simulink model "BSPK_Sound"  (R2024b)
settings: Solver=VariableStepAuto  StartTime=0.0  StopTime=5.5  RelTol=1e-3
libraries: commdigbbndpm3 x2, simulink x2, commchan3 x1, commsink2 x1, dspvision x1, dspsnks4 x1
settings Model: Creator=sarriola  LastModifiedBy=RomaW11
settings SolverCC: AlgebraicLoopSolver=TrustRegion
settings DataIOCC: ReturnWorkspaceOutputs=off
settings OptimizationCC: LifeSpan=inf
settings DebuggingCC: UnconnectedInputMsg=warning  UnconnectedOutputMsg=warning  UnconnectedLineMsg=warning  SFExecutionAtInitializationDiag=none  ArithmeticOperatorsInVariantConditions=warning
settings ModelReferenceCC: EnableRefExpFcnMdlSchedulingChecks=on
settings SFSimCC: SimUseLocalCustomCode=off  CustomCodeUndefinedFunction=UseInterfaceOnly
settings RTWCC: RTWUseLocalCustomCode=off  GPUComputeCapability=3.5
settings CodeAppCC: StateflowObjectComments=on

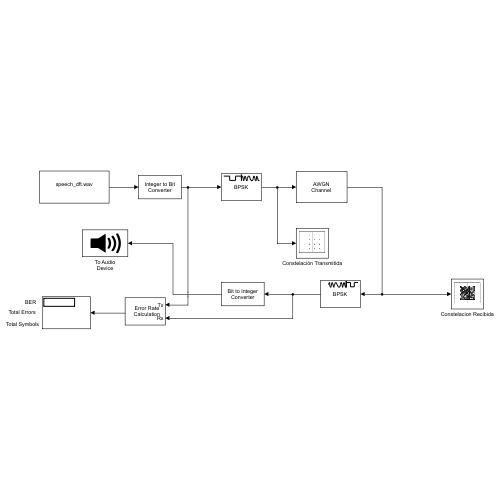
[thumbnail: Simulink's stored preview of the top-level diagram]
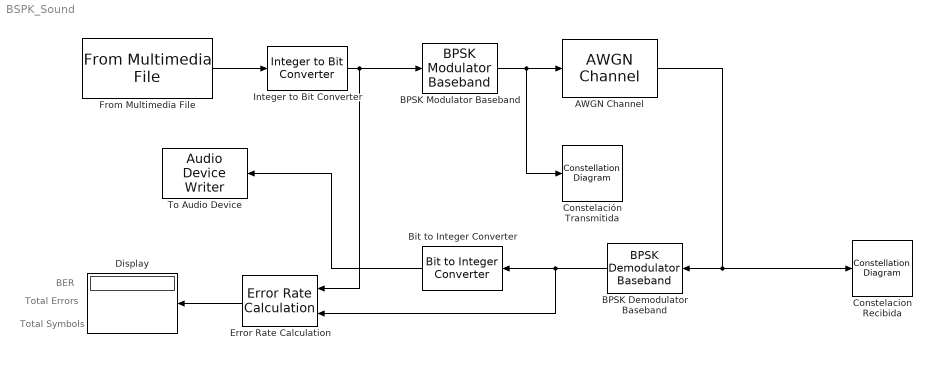
== system BSPK_Sound ==
  note: Total Symbols
  note: Total Errors
  note: BER
  AWGN Channel : commchan3/AWGN Channel  LegacyMode=on  NoiseMethod="Signal to noise ratio  (SNR)"  noiseMode="Signal to noise ratio  (SNR)"  EbNo=60  EsNo=10  SNR=30  BitsPerSymbol=1  SignalPower=1  SamplesPerSymbol=1  SymbolPeriod=1  VarianceSource=Parameter  Variance=1  RandomStream=Global stream  Seed=67  SimulateUsing=Code generation
  BPSK Demodulator Baseband : commdigbbndpm3/BPSK Demodulator Baseband  DecType=Hard decision  VarSource=Dialog  Variance=1  Ph=0  outDtype=int16  derotateFactorWordLen=16  derotateFactorDataTypeStr=Inherit: Same word length as input  derotateFactorLastDataTypeStr=Inherit: Same word length as input
  BPSK Modulator Baseband : commdigbbndpm3/BPSK Modulator Baseband  Ph=0  outDtype=double  outWordLen=16  outUDDataType=sfix(16)  outFracLenMode=Best precision  outFracLen=15  outDataTypeStr=double  outLastDataTypeStr=double
  Bit to Integer Converter : simulink/Logic and Bit Operations/Bit to Integer Converter  nbits=16  bitOrder=MSB first  signedOutputValues=Signed  outDtype=int16  outDtypeSigned=int16
      settings: LibrarySourceBlock=|
      | commutil2/Bit to Integer
      | Converter
  "Constelacion Recibida " : ConstellationDiagram  WindowPosition=[513 212 341 345]  ShowTrajectory=on  DefaultConfigurationName=comm.scopes.ConstellationDiagramBlockCfg
  "Constelación Transmitida " : ConstellationDiagram  WindowPosition=[873 209 341 345]  ShowTrajectory=on  DefaultConfigurationName=comm.scopes.ConstellationDiagramBlockCfg
  Display : Display
  Error Rate Calculation : commsink2/Error Rate Calculation  N=0  st_delay=0  cp_mode=Entire frame  subframe=[]  PMode=Port  WsName=ErrorVec  RsMode2=off  stop=off  numErr=100  maxBits=1e6
  From Multimedia File : dspvision/From Multimedia File  inputFilename=D:\Semestre 2020\TEC\2020\I Semestre\Taller de Comunicaciones Eléctricas\Instructivos Laboratorio\Virtual\Laboratorio 4\Practica\Simulink\speech_dft.wav  readRange=[1 Inf]  loop=on  numPlays=inf  outputStreams=Audio only  videoDataType=single  audioDataType=int16  inheritSampleTime=on  userDefinedSampleTime=1/30  noAudioOutput=off  isIntensityVideo=off  fourcc=RGB  colorVideoFormat=Separate color signals  outputEOF=off  dataOrg=Column-major  audioFrameSize=1024  computeAudioFrameSize=off  outSamplingMode=Sample based
  Integer to Bit Converter : simulink/Logic and Bit Operations/Integer to Bit Converter  nbits=16  signedInputValues=Signed  bitOrder=MSB first  outDtype=int16
      settings: LibrarySourceBlock=|
      | commutil2/Integer to Bit
      | Converter
  To Audio Device : dspsnks4/Audio Device Writer  Driver=DirectSound  Device=Default  InheritSampleRate=on  SampleRate=44100  BitDepth=16-bit integer  BufferSize=4096  NumBuffers=10  DefaultOutputChannelMapping=on  OutputChannelMapping=1:2  OutputNumUnderrunSamples=off  DriverIdx=1  DeviceWarnFlag=''
  wires:
  AWGN Channel/1 -> BPSK Demodulator Baseband/1, "Constelacion Recibida "/1
  BPSK Demodulator Baseband/1 -> Error Rate Calculation/2, Bit to Integer Converter/1
  From Multimedia File/1 -> Integer to Bit Converter/1
  Integer to Bit Converter/1 -> BPSK Modulator Baseband/1, Error Rate Calculation/1
  BPSK Modulator Baseband/1 -> "Constelación Transmitida "/1, AWGN Channel/1
  Bit to Integer Converter/1 -> To Audio Device/1
  Error Rate Calculation/1 -> Display/1
